simulink model "basic_model"  (R2020a)
settings: Solver=ode45  StartTime=0.0  StopTime=10.0  RelTol=1e-9  AbsTol=1e-10
PreLoadFcn:
  | model_startup
settings Model: Creator=Justi  LastModifiedBy=Justi

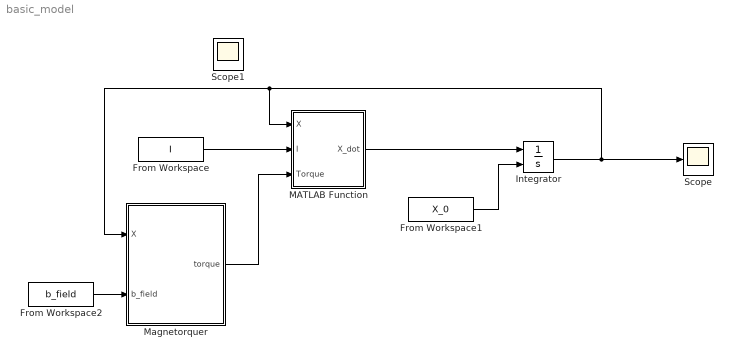
== system basic_model ==
  From Workspace : FromWorkspace  VariableName=I
  From Workspace1 : FromWorkspace  VariableName=X_0
  From Workspace2 : FromWorkspace  VariableName=b_field
  Integrator : Integrator  InitialConditionSource=external  AbsoluteTolerance=0.000000001  ZeroCross=off
  MATLAB Function : MATLAB Function  TreatAsAtomicUnit=on
  "Magnetorquer " : MATLAB Function  TreatAsAtomicUnit=on
  Scope : Scope
  Scope1 : Scope
  wires:
  MATLAB Function/1(X_dot) -> Integrator/1
  Integrator/1 -> "Magnetorquer "/1(X), MATLAB Function/1(X), Scope/1
  From Workspace1/1 -> Integrator/2
  From Workspace/1 -> MATLAB Function/2(I)
  "Magnetorquer "/1(torque) -> MATLAB Function/3(Torque)
  From Workspace2/1 -> "Magnetorquer "/2(b_field)

== matlab function basic_model/MATLAB Function ==
  data: X input; X_dot output; I input; Torque input
function X_dot = EOM(X,I,Torque)
Ix = I(1,1);
Iy = I(2,2);
Iz = I(3,3);
X_dot = EOMS(0,X,Ix,Iy,Iz,Torque);

== matlab function basic_model/Magnetorquer  ==
  data: X input; torque output; b_field input
function torque = torque_imparted(X,b_field)

torque = zeros(3,1);

euler_params = X(1:4);

%Covering each magnetorquer 
for i = 1:3
    torque(i) = magnetorquer(b_field,i,euler_params);
end

end
